simulink model "hiperlan2"  (Simulink 6.0)
settings: Solver=FixedStepDiscrete  SolverMode=SingleTasking  StartTime=0.0  StopTime=250  RelTol=1e-3
undefined symbols (not defined in the file or in its folder): figposition, Fs, slcm
libraries: commblkintrlv2 x4, commsink2 x3, commcnvcod2 x2, commsequence2 x2, dspxfrm3 x2, dspindex x2, commutil2 x2, commdigbbndam2 x2, commchan2 x1, commrandsrc2 x1, dspsigattribs x1, dspsrcs4 x1
CloseFcn:
  | clear hlanSigsOut
settings Model: Creator=mclune  LastModifiedBy=arodrigu  ExtModeAutoUpdateStatusClock=off
settings DataIOCC: LimitDataPoints=off  SaveOutput=off  SaveTime=off  SignalLoggingName=hlanSigsOut
settings OptimizationCC: BooleanDataType=off
settings DebuggingCC: CheckExecutionContextPreStartOutputMsg=on  CheckExecutionContextRuntimeOutputMsg=on  SolverPrmCheckMsg=none  InheritedTsInSrcMsg=none
settings HardwareCC: TargetUnknown=on
settings ModelReferenceCC: UpdateModelReferenceTargets=IfOutOfDate

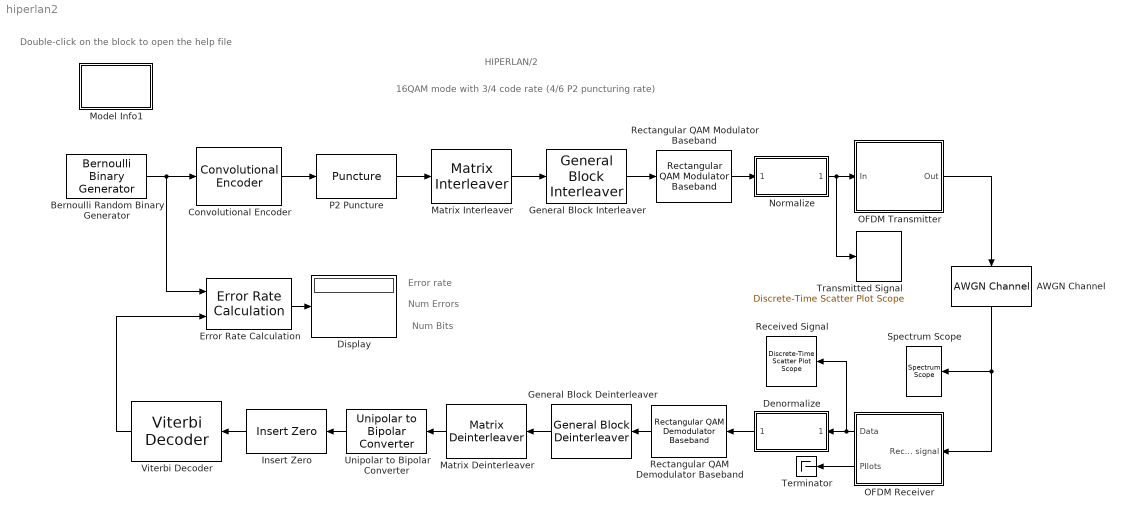
== system hiperlan2 ==
  note: HIPERLAN/2
  note: Error rate
  note: Num Errors
  note: Num Bits
  note: 16QAM mode with 3/4 code rate (4/6 P2 puncturing rate)
  note: Double-click on the block
      | to open the help file
  AWGN Channel : commchan2/AWGN Channel  Orientation=down  seed=1  noiseMode="Signal to noise ratio  (SNR)"  EbNodB=10  EsNodB=40  SNRdB=15  bitsPerSym=1  Ps=0.01  Tsym=4e-6/80  variance=1
  Bernoulli Random Binary Generator : commrandsrc2/Bernoulli Binary Generator  P=0.5  seed=20394875  Ts=4e-6/144  frameBased=on  sampPerFrame=144  orient=off
  Convolutional Encoder : commcnvcod2/Convolutional Encoder  trellis=poly2trellis(7, [133 171])  reset=None
  Denormalize : Subsystem  Orientation=left  PropExecContextAcrossSSBoundary=on
      mask Display: disp('Denormalize');
  Display : Display
  Error Rate Calculation : commsink2/Error Rate Calculation  N=34  st_delay=0  cp_mode=Entire frame  subframe=[]  PMode=Port  WsName=ErrorVec  RsMode2=off  stop=off  numErr=100  maxBits=1e6
  General Block Deinterleaver : commblkintrlv2/General Block Deinterleaver  Orientation=left  elements=[ 2*floor( [0:191]/2 ) + mod( ([0:191] + 192 - floor( 16*[0:191]/192 ) ) ,2 ) + 1]'
  General Block Interleaver : commblkintrlv2/General Block Interleaver  elements=[ 2*floor( [0:191]/2 ) + mod( ([0:191] + 192 - floor( 16*[0:191]/192 ) ) ,2 ) + 1]'
  Insert Zero : commsequence2/Insert Zero  Orientation=left  insertZeroVector=[1 1 1 0 0 1]'
  Matrix Deinterleaver : commblkintrlv2/Matrix Deinterleaver  Orientation=left  Nrows=16  Ncols=12
  Matrix Interleaver : commblkintrlv2/Matrix Interleaver  Nrows=16  Ncols=12
  Model Info1 : Subsystem  LoadFcn=slcm LoadBlock;  InitFcn=slcm('UpdateAllCMBlocksInThisModelInit')  PropExecContextAcrossSSBoundary=on  mask(CMBlock){InitialSaveTempField=, InitialBlockCM=None, BlockCM=None, Frame=on, SaveTempField=, DisplayStringWithTags=Info, MaskDisplayString=Info, HorizontalTextAlignment=Center, LeftAlignmentValue=0.5, SourceBlockDiagram=hiperlan2, TagMaxNumber=20, CMTag1=, CMTag2=, CMTag3=, CMTag4=, CMTag5=, CMTag6=, CMTag7=, CMTag8=, CMTag9=, CMTag10=, CMTag11=, CMTag12=, CMTag13=, CMTag14=, CMTag15=, CMTag16=, CMTag17=, CMTag18=, CMTag19=, CMTag20=}
      mask help: This block allows revision control information to be displayed within the model.
      settings: CopyFcn=slcm CopyBlock;  DeleteFcn=slcm Cancel;  PostSaveFcn=slcm('UpdateAllCMBlocksInThisModel')  NameChangeFcn=slcm Rename;  OpenFcn=commdemohelp;
      mask Display: text(str2num(LeftAlignmentValue), 0.5, MaskDisplayString, 'HorizontalAlignment', HorizontalTextAlignment)
  Normalize : Subsystem  PropExecContextAcrossSSBoundary=on
      mask Display: disp('Normalize')
  OFDM Receiver : Subsystem  Orientation=left  PropExecContextAcrossSSBoundary=on
      mask Display:
      | disp('OFDM\nReceiver');
      | port_label('output',2,'pilots')
  OFDM Transmitter : Subsystem  PropExecContextAcrossSSBoundary=on
      mask Display: disp('OFDM\nTransmitter')
  P2 Puncture : commsequence2/Puncture  punctureVector=[1 1 1 0 0 1]'
  Received Signal : commsink2/Discrete-Time Scatter Plot Scope  Tag=ScatterPlot  Orientation=left  sampPerSymb=1  offsetEye=0  numTraces=160  numNewFrames=80  LineMarkers=.  LineColors=b  fading=on  render=off  AxisGrid=on  xMin=-1.5  xMax=1.5  yMin=-1.5  yMax=1.5  inphaseLabel=In-phase Amplitude  quadratureLabel=Quadrature Amplitude  openScopeAtSimStart=on  FrameNumber=off  FigPos="figposition([54    51    35    40])"  figTitle=Scatter Plot  numLinesMax=8  block_type_=scatter
  Rectangular QAM Demodulator Baseband : commdigbbndam2/Rectangular QAM Demodulator Baseband  Orientation=left  M=16  OutType=Bit  Dec=Gray  PowType=Min. distance between symbols  MinDist=2  AvgPow=1  PeakPow=1  Ph=0  numSamp=1
  Rectangular QAM Modulator Baseband : commdigbbndam2/Rectangular QAM Modulator Baseband  M=16  InType=Bit  Enc=Gray  PowType=Min. distance between symbols  MinDist=2  AvgPow=1  PeakPow=1  Ph=0  numSamp=1
  Spectrum Scope : dspsnks4/Spectrum Scope  Orientation=left  ScopeProperties=off  Domain=Frequency  HorizSpan=1  UseBuffer=on  BufferSize=80  Overlap=0  inpFftLenInherit=on  FFTlength=1024  numAvg=10  DisplayProperties=off  AxisGrid=on  Memory=off  FrameNumber=on  AxisLegend=off  AxisZoom=off  OpenScopeAtSimStart=on  OpenScopeImmediately=off  FigPos="figposition([25    15    42    27])"  AxisProperties=off  XUnits=Hertz  XRange=[-Fs/2...Fs/2]  InheritXIncr=off  XIncr=1.0  XLabel=Samples  YUnits=dB  YLabel=Magnitude, dB  LineProperties=off
      settings: YMin=-60  YMax=0
  Terminator : Terminator
  Transmitted Signal : commsink2/Discrete-Time Scatter Plot Scope  Tag=ScatterPlot  sampPerSymb=1  offsetEye=0  numTraces=60  numNewFrames=60  LineMarkers=.  LineColors=r  fading=off  render=on  AxisGrid=on  xMin=-1.5  xMax=1.5  yMin=-1.5  yMax=1.5  inphaseLabel=In-phase Amplitude  quadratureLabel=Quadrature Amplitude  openScopeAtSimStart=on  FrameNumber=off  FigPos="figposition([7    51    35    40])"  figTitle=Scatter Plot  numLinesMax=8  block_type_=scatter
  Unipolar to Bipolar Converter : commutil2/Unipolar to Bipolar Converter  Orientation=left  M=2  polarity=Negative
  Viterbi Decoder : commcnvcod2/Viterbi Decoder  Orientation=left  trellis=poly2trellis(7, [133 171])  dectype=Unquantized  nsdecb=4  tbdepth=34  opmode=Continuous  reset=off
  wires:
  Rectangular QAM Modulator Baseband/1 -> Normalize/1("   ")
  Bernoulli Random Binary Generator/1 -> Convolutional Encoder/1, Error Rate Calculation/1
  OFDM Transmitter/1(Out) -> AWGN Channel/1
  Viterbi Decoder/1 -> Error Rate Calculation/2
  P2 Puncture/1 -> Matrix Interleaver/1
  General Block Interleaver/1 -> Rectangular QAM Modulator Baseband/1
  General Block Deinterleaver/1 -> Matrix Deinterleaver/1
  Convolutional Encoder/1 -> P2 Puncture/1
  Insert Zero/1 -> Viterbi Decoder/1
  Matrix Deinterleaver/1 -> Unipolar to Bipolar Converter/1
  Rectangular QAM Demodulator Baseband/1 -> General Block Deinterleaver/1
  Normalize/1("  ") -> OFDM Transmitter/1(In), Transmitted Signal/1
  Denormalize/1("  ") -> Rectangular QAM Demodulator Baseband/1
  Unipolar to Bipolar Converter/1 -> Insert Zero/1
  OFDM Receiver/1(Data) -> Denormalize/1("   "), Received Signal/1
  Error Rate Calculation/1 -> Display/1
  AWGN Channel/1 -> OFDM Receiver/1(Received signal), Spectrum Scope/1
  Matrix Interleaver/1 -> General Block Interleaver/1
  OFDM Receiver/2(PIlots) -> Terminator/1

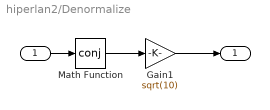
== system hiperlan2/Denormalize ==
  "   " : Inport  LatchInput=off
  Gain1 : Gain  Gain=sqrt(10)  SaturateOnIntegerOverflow=on
  Math Function : Math  Operator=conj  SaturateOnIntegerOverflow=on
  "  " : Outport
  wires:
  "   "/1 -> Math Function/1
  Math Function/1 -> Gain1/1
  Gain1/1 -> "  "/1

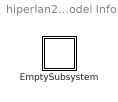
== system hiperlan2/Model Info1 ==
  EmptySubsystem : Subsystem  PropExecContextAcrossSSBoundary=on

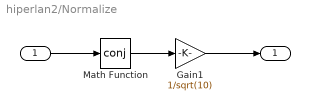
== system hiperlan2/Normalize ==
  "   " : Inport  LatchInput=off
  Gain1 : Gain  Gain=1/sqrt(10)  SaturateOnIntegerOverflow=on
  Math Function : Math  Operator=conj  SaturateOnIntegerOverflow=on
  "  " : Outport
  wires:
  Math Function/1 -> Gain1/1
  "   "/1 -> Math Function/1
  Gain1/1 -> "  "/1

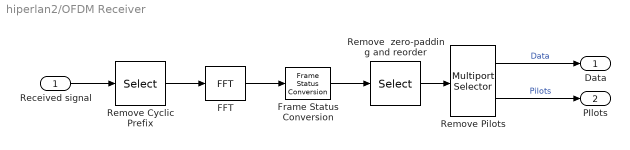
== system hiperlan2/OFDM Receiver ==
  Received signal : Inport  LatchInput=off
  FFT : dspxfrm3/FFT  CompMethod=Table lookup  TableOpt=Speed  BitRevOrder=off  SkipNorm=off  firstCoeffMode=User-defined  firstCoeffWordLength=16  firstCoeffFracLength=15  roundingMode=Floor  overflowMode=off
  Frame Status Conversion : dspsigattribs/Frame Status Conversion  growRefPort=off  outframe=Frame-based
  Remove  zero-padding and reorder : Selector  Elements=[39:64 1:27]  InputPortWidth=64
  Remove Pilots : dspindex/Multiport Selector  rowsOrCols=Rows  idxCellArray={[1:5 7:19 21:26 28:33 35:47 49:53],[6 20 34 48]}  idxErrMode=Clip Index
  Remove Cyclic Prefix : Selector  Elements=[17:80]  InputPortWidth=80
  Data : Outport
  PIlots : Outport  Port=2
  wires:
  Frame Status Conversion/1 -> Remove  zero-padding and reorder/1
  FFT/1 -> Frame Status Conversion/1
  Received signal/1 -> Remove Cyclic Prefix/1
  Remove Cyclic Prefix/1 -> FFT/1
  Remove  zero-padding and reorder/1 -> Remove Pilots/1
  Remove Pilots/1 -> Data/1  "Data"
  Remove Pilots/2 -> PIlots/1  "Pilots"

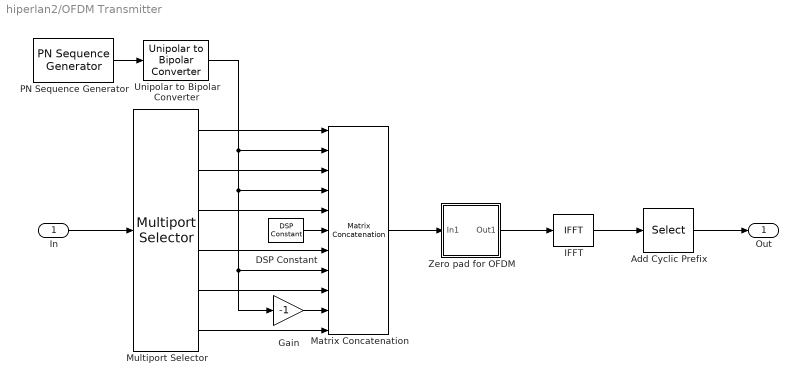
== system hiperlan2/OFDM Transmitter ==
  In : Inport  LatchInput=off
  Add Cyclic Prefix : Selector  Elements=[49:64 1:64]  InputPortWidth=64
  DSP Constant : dspsrcs4/DSP Constant  Value=0+0i  SampleMode=Discrete  discreteOutput=Frame-based  continuousOutput=Sample-based  sampTime=4e-6  framePeriod=4e-6  dataType=Inherit from 'Constant value'  wordLen=16  udDataType=sfix(16)  fracBitsMode=Best precision  numFracBits=15  InterpretAs1D=off  Ts=4e-6  FramebasedOutput=on
  Gain : Gain  Gain=-1  SaturateOnIntegerOverflow=on
  IFFT : dspxfrm3/IFFT  CompMethod=Table lookup  TableOpt=Speed  BitRevOrder=off  cs_in=off  SkipNorm=off  mode=Complex  firstCoeffMode=User-defined  firstCoeffWordLength=16  firstCoeffFracLength=15  roundingMode=Floor  overflowMode=off
  Matrix Concatenation : simulink/Math Operations/Matrix Concatenation  numInports=11  catMethod=Vertical
  Multiport Selector : dspindex/Multiport Selector  rowsOrCols=Rows  idxCellArray={1:5,6:18,19:24,25:30,31:43,44:48}  idxErrMode=Clip Index
  PN Sequence Generator : commseqgen2/PN Sequence Generator  poly=[1 0 0 1 0 0 0 1]  ini_sta=[1 1 1 1 1 1 1]  shift=0  Ts=4e-6  frameBased=off  sampPerFrame=1  reset=off
  Unipolar to Bipolar Converter : commutil2/Unipolar to Bipolar Converter  M=2  polarity=Negative
  Zero pad for OFDM : Subsystem  PropExecContextAcrossSSBoundary=on
      mask Display: disp('Zero pad\nfor OFDM');
  Out : Outport
  wires:
  Zero pad for OFDM/1(Out1) -> IFFT/1
  IFFT/1 -> Add Cyclic Prefix/1
  Add Cyclic Prefix/1 -> Out/1
  PN Sequence Generator/1 -> Unipolar to Bipolar Converter/1
  Unipolar to Bipolar Converter/1 -> Matrix Concatenation/2, Matrix Concatenation/4, Matrix Concatenation/8, Gain/1
  Matrix Concatenation/1 -> Zero pad for OFDM/1(In1)
  DSP Constant/1 -> Matrix Concatenation/6
  Multiport Selector/1 -> Matrix Concatenation/1
  Multiport Selector/2 -> Matrix Concatenation/3
  Multiport Selector/3 -> Matrix Concatenation/5
  Multiport Selector/4 -> Matrix Concatenation/7
  Multiport Selector/5 -> Matrix Concatenation/9
  Multiport Selector/6 -> Matrix Concatenation/11
  Gain/1 -> Matrix Concatenation/10
  In/1 -> Multiport Selector/1

== system hiperlan2/Model Info1/EmptySubsystem ==

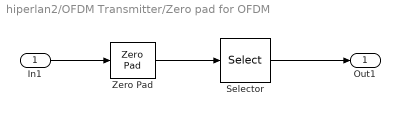
== system hiperlan2/OFDM Transmitter/Zero pad for OFDM ==
  In1 : Inport  LatchInput=off
  Selector : Selector  Elements=[27:64 1:26]  InputPortWidth=64
  Zero Pad : dspsigops/Zero Pad  padSigAt=End  zpadAlong=Columns  padNumOutRowsSpecMethod=User-specified  numOutRows=64  padNumOutColsSpecMethod=User-specified  numOutCols=1  trunc_flag=None
  Out1 : Outport
  wires:
  Selector/1 -> Out1/1
  Zero Pad/1 -> Selector/1
  In1/1 -> Zero Pad/1
